simulink model "mbs"  (R2024a)
settings: Solver=VariableStepAuto  StartTime=0.0  StopTime=10.0  RelTol=1e-3
settings Model: Creator=mrvol  LastModifiedBy=mrvol

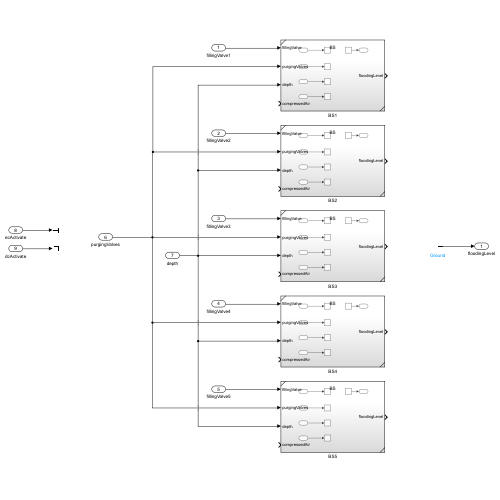
[thumbnail: Simulink's stored preview of the top-level diagram]
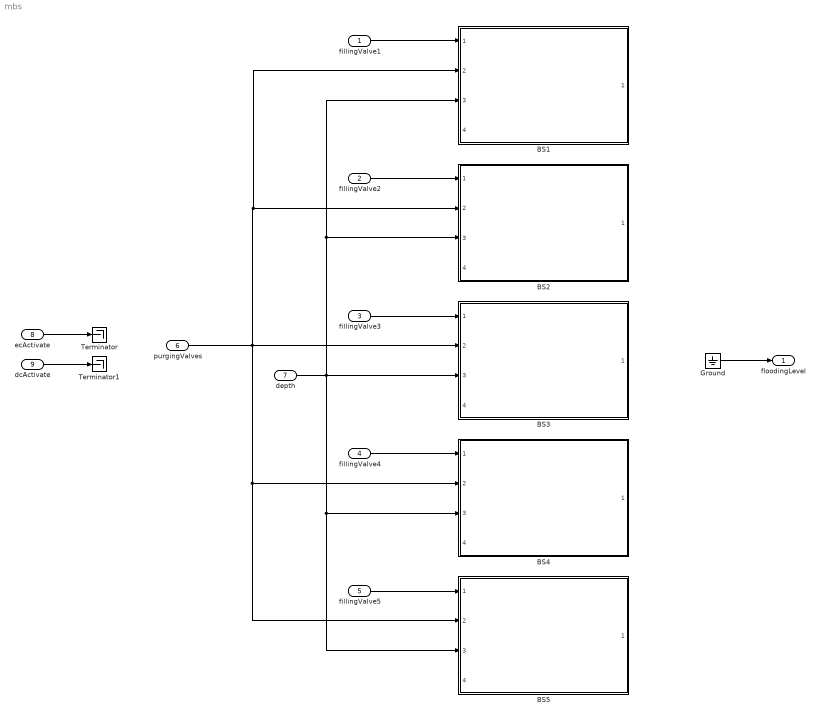
== system mbs ==
  fillingValve1 : Inport
  fillingValve2 : Inport  Port=2
  fillingValve3 : Inport  Port=3
  fillingValve4 : Inport  Port=4
  fillingValve5 : Inport  Port=5
  purgingValves : Inport  Port=6
  depth : Inport  Port=7
  ecActivate : Inport  Port=8
  dcActivate : Inport  Port=9
  BS{1..5} (5 alike) : Subsystem  ReferencedSubsystem=BS
  Ground : Ground
  Terminator : Terminator
  Terminator1 : Terminator
  floodingLevel : Outport
  wires:
  depth/1 -> BS4/3, BS5/3, BS1/3, BS2/3, BS3/3
  fillingValve1/1 -> BS1/1
  fillingValve2/1 -> BS2/1
  fillingValve3/1 -> BS3/1
  fillingValve4/1 -> BS4/1
  fillingValve5/1 -> BS5/1
  purgingValves/1 -> BS3/2, BS1/2, BS2/2, BS5/2, BS4/2
  ecActivate/1 -> Terminator/1
  dcActivate/1 -> Terminator1/1
  Ground/1 -> floodingLevel/1
